simulink model "Dead_Zone_verif"  (Simulink 7.2)
settings: Solver=ode45  StartTime=0.0  StopTime=10.0  RelTol=1e-3
undefined symbols (not defined in the file): sample
settings Model: Creator=Romain  LastModifiedBy=Romain
settings OptimizationCC: ExpressionDepthLimit=128
settings DebuggingCC: SolverPrmCheckMsg=none  FcnCallInpInsideContextMsg=Enable All  StateNameClashWarn=none  StrictBusMsg=ErrorLevel1
settings CodeAppCC: CustomSymbolStrType=$N$R$M_T
settings GRTTargetCC: TargetFunctionLibrary=C89/C90 (ANSI)

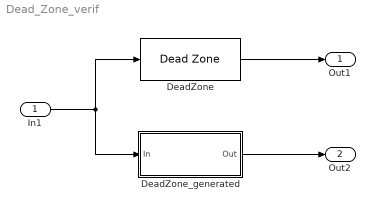
== system Dead_Zone_verif ==
  In1 : Inport  OutDataTypeStr=double  DataType=double
  DeadZone : DeadZone  SaturateOnIntegerOverflow=on
  DeadZone_generated : Subsystem  TreatAsAtomicUnit=on
  Out1 : Outport
  Out2 : Outport  Port=2
  wires:
  In1/1 -> DeadZone_generated/1(In), DeadZone/1
  DeadZone/1 -> Out1/1
  DeadZone_generated/1(Out) -> Out2/1

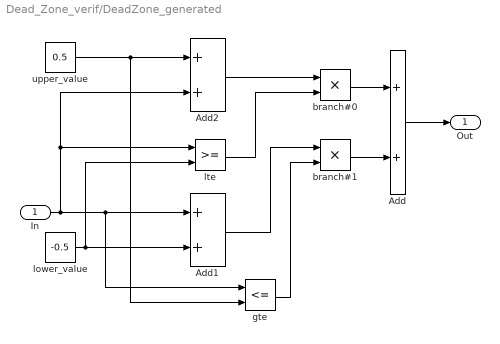
== system Dead_Zone_verif/DeadZone_generated ==
  In : Inport
  Add : Sum
  Add1 : Sum
  Add2 : Sum
  branch#0 : Product  RndMeth=Zero
  branch#1 : Product  RndMeth=Zero
  gte : RelationalOperator  Operator=<=  OutDataTypeStr=boolean  SampleTime=sample  LogicOutDataTypeMode=boolean
  lower_value : Constant  Value=-0.5  SampleTime=sample
  lte : RelationalOperator  OutDataTypeStr=boolean  LogicOutDataTypeMode=boolean
  upper_value : Constant  Value=0.5  SampleTime=sample
  Out : Outport
  wires:
  In/1 -> Add1/1, gte/1, Add2/2, lte/1
  lower_value/1 -> Add1/2, lte/2
  Add/1 -> Out/1
  upper_value/1 -> Add2/1, gte/2
  Add2/1 -> branch#0/1
  branch#0/1 -> Add/1
  lte/1 -> branch#0/2
  Add1/1 -> branch#1/1
  gte/1 -> branch#1/2
  branch#1/1 -> Add/2
